simulink model "W15_Road_Side_Parking_cs"  (R2019a)
settings: Solver=ode5  StartTime=0.0  StopTime=inf  FixedStep=1/20  RelTol=1e-3
PreLoadFcn:
  | mbxruntime.callbacks.PreLoadFcn(bdroot);
PostLoadFcn:
  | mbxruntime.callbacks.PostLoadFcn(bdroot);
InitFcn:
  | mbxruntime.callbacks.InitFcn(bdroot);
StartFcn:
  | mbxruntime.callbacks.StartFcn(bdroot);
StopFcn:
  | mbxruntime.callbacks.StopFcn(bdroot);
model workspace: external: MAT-File .\W15_Road_Side_Parking_cs_hws.mat (data not in the file)
undefined symbols (not defined in the file or in its folder): DiscIntNeverNeededParam, mbxruntime, W15_Road_Side_Parking_cs_0e866b970dd74d99, W15_Road_Side_Parking_cs_0f148a56f75f3276, W15_Road_Side_Parking_cs_17cd01741fd6f084, W15_Road_Side_Parking_cs_18be040ea5165f26, W15_Road_Side_Parking_cs_18f6c04aadf175ba, W15_Road_Side_Parking_cs_1923d3106c1c637d, W15_Road_Side_Parking_cs_1b5a4544d45624a7, W15_Road_Side_Parking_cs_1b6c0c20ec73a43a, W15_Road_Side_Parking_cs_2b0ebcffe59377d8, W15_Road_Side_Parking_cs_31ff6997c9af0f31, W15_Road_Side_Parking_cs_38fd1df42ec62113, W15_Road_Side_Parking_cs_3b33461cc0923d5a, W15_Road_Side_Parking_cs_3fb29b605fd2446e, W15_Road_Side_Parking_cs_415727a4762a2f3b, W15_Road_Side_Parking_cs_42e4989f077d83f1, W15_Road_Side_Parking_cs_437d21a73ee2a604, W15_Road_Side_Parking_cs_438c4f208d99b00a, W15_Road_Side_Parking_cs_43af58d29723f162, W15_Road_Side_Parking_cs_46e56dcb0f84eb7a, W15_Road_Side_Parking_cs_4b469b712dfdc78c, W15_Road_Side_Parking_cs_52f5bda9b370cee6, W15_Road_Side_Parking_cs_53d6cec13a681255, W15_Road_Side_Parking_cs_55198fcb4bd3c3cf, W15_Road_Side_Parking_cs_55651d2ac6314b5a, W15_Road_Side_Parking_cs_566668cc8d93055a, W15_Road_Side_Parking_cs_5685e0897f4c48c1, W15_Road_Side_Parking_cs_59579d35ff31c10a, W15_Road_Side_Parking_cs_59ff7782c70c6b28, W15_Road_Side_Parking_cs_5bf98cb8ec781366, W15_Road_Side_Parking_cs_5f42887855dc872c, W15_Road_Side_Parking_cs_6189064c2a21a5a0, W15_Road_Side_Parking_cs_6a2215e73604bb67, W15_Road_Side_Parking_cs_71a8b3b44613f615, W15_Road_Side_Parking_cs_71c6ac7bb3dca246, W15_Road_Side_Parking_cs_71fd76710240543d, W15_Road_Side_Parking_cs_745c3945ff638ec3, W15_Road_Side_Parking_cs_7a6c1e7b0eb6c7b9, W15_Road_Side_Parking_cs_85e359d40c717561, W15_Road_Side_Parking_cs_8b52fd1869158bfe, W15_Road_Side_Parking_cs_8bff9458d942351f, W15_Road_Side_Parking_cs_8c4b607c5829f2a9, W15_Road_Side_Parking_cs_8f8185f5cf144aaf, W15_Road_Side_Parking_cs_93695886b652e87b, W15_Road_Side_Parking_cs_97c6d597a0216a81, W15_Road_Side_Parking_cs_9b084c5c3aa0b401, W15_Road_Side_Parking_cs_9c145665a20a76f3, W15_Road_Side_Parking_cs_9dd5e77a4f43e96a, W15_Road_Side_Parking_cs_a44a67f2721d9815, W15_Road_Side_Parking_cs_a5d6455b7e6bd0b2, W15_Road_Side_Parking_cs_a72a872bc8c596f9, W15_Road_Side_Parking_cs_ab6502bd2087c801, W15_Road_Side_Parking_cs_ad8c05542c501359, W15_Road_Side_Parking_cs_ae0701bb52210b9e, W15_Road_Side_Parking_cs_b19e05410c02f142, W15_Road_Side_Parking_cs_b31b08a7b69b63e6, W15_Road_Side_Parking_cs_b3b5053d85c8642b, W15_Road_Side_Parking_cs_bbd847625a8d6d3d, W15_Road_Side_Parking_cs_bc9116e6f1ce847b ... (+26)
libraries: adeye_lib x37, PreScanSimulinkLibrary x28, PreScanUsefulBlocks x1
(part 2 of 10)

== system W15_Road_Side_Parking_cs/AIR_3 ==
  Sensor : S-Function  FunctionName=sfun_AIRSensor  Parameters=mbxruntime.parameters.convert(detectableObjects), mbxruntime.parameters.convert(sensorID), mbxruntime.parameters.convert(timestep)  SFunctionDeploymentMode=off  EnableBusSupport=off  mask(PreScan Source Block: Actor Independent Receiver (AIR)){detectableObjects=1, sensorID=3596, timestep=1/20}
      mask prompts: detectableObjects "Max detectable objects"; sensorID "Sensor ID"; timestep "MATLAB timestep:"
      mask help:
      | The Actor Information Receiver sensor provides a fast, simple and generic detection solution which is not tied up to a specific technology. The AIR detects the intersection point of the bounding box with the straight line from the sensor axis system to the middle of the bounding box.
      |
      | For more information, please click Help.
      mask Help: eval('openHelp(413)')
      mask Display: image(imread('AIR.png'))
  AIR_3 : Outport  Tag=outport/AIR  OutDataTypeStr=Bus: PRESCAN_AIRSENSORMESSAGE  PortDimensions=1  SampleTime=1/20
  wires:
  Sensor/1 -> AIR_3/1

== system W15_Road_Side_Parking_cs/AIR_4 ==
  Sensor : S-Function  FunctionName=sfun_AIRSensor  Parameters=mbxruntime.parameters.convert(detectableObjects), mbxruntime.parameters.convert(sensorID), mbxruntime.parameters.convert(timestep)  SFunctionDeploymentMode=off  EnableBusSupport=off  mask(PreScan Source Block: Actor Independent Receiver (AIR)){detectableObjects=1, sensorID=3598, timestep=1/20}
      mask prompts: detectableObjects "Max detectable objects"; sensorID "Sensor ID"; timestep "MATLAB timestep:"
      mask help:
      | The Actor Information Receiver sensor provides a fast, simple and generic detection solution which is not tied up to a specific technology. The AIR detects the intersection point of the bounding box with the straight line from the sensor axis system to the middle of the bounding box.
      |
      | For more information, please click Help.
      mask Help: eval('openHelp(413)')
      mask Display: image(imread('AIR.png'))
  AIR_4 : Outport  Tag=outport/AIR  OutDataTypeStr=Bus: PRESCAN_AIRSENSORMESSAGE  PortDimensions=1  SampleTime=1/20
  wires:
  Sensor/1 -> AIR_4/1

== system W15_Road_Side_Parking_cs/AIR_5 ==
  Sensor : S-Function  FunctionName=sfun_AIRSensor  Parameters=mbxruntime.parameters.convert(detectableObjects), mbxruntime.parameters.convert(sensorID), mbxruntime.parameters.convert(timestep)  SFunctionDeploymentMode=off  EnableBusSupport=off  mask(PreScan Source Block: Actor Independent Receiver (AIR)){detectableObjects=1, sensorID=3600, timestep=1/20}
      mask prompts: detectableObjects "Max detectable objects"; sensorID "Sensor ID"; timestep "MATLAB timestep:"
      mask help:
      | The Actor Information Receiver sensor provides a fast, simple and generic detection solution which is not tied up to a specific technology. The AIR detects the intersection point of the bounding box with the straight line from the sensor axis system to the middle of the bounding box.
      |
      | For more information, please click Help.
      mask Help: eval('openHelp(413)')
      mask Display: image(imread('AIR.png'))
  AIR_5 : Outport  Tag=outport/AIR  OutDataTypeStr=Bus: PRESCAN_AIRSENSORMESSAGE  PortDimensions=1  SampleTime=1/20
  wires:
  Sensor/1 -> AIR_5/1

== system W15_Road_Side_Parking_cs/AIR_6 ==
  Sensor : S-Function  FunctionName=sfun_AIRSensor  Parameters=mbxruntime.parameters.convert(detectableObjects), mbxruntime.parameters.convert(sensorID), mbxruntime.parameters.convert(timestep)  SFunctionDeploymentMode=off  EnableBusSupport=off  mask(PreScan Source Block: Actor Independent Receiver (AIR)){detectableObjects=1, sensorID=3960, timestep=1/20}
      mask prompts: detectableObjects "Max detectable objects"; sensorID "Sensor ID"; timestep "MATLAB timestep:"
      mask help:
      | The Actor Information Receiver sensor provides a fast, simple and generic detection solution which is not tied up to a specific technology. The AIR detects the intersection point of the bounding box with the straight line from the sensor axis system to the middle of the bounding box.
      |
      | For more information, please click Help.
      mask Help: eval('openHelp(413)')
      mask Display: image(imread('AIR.png'))
  AIR_6 : Outport  Tag=outport/AIR  OutDataTypeStr=Bus: PRESCAN_AIRSENSORMESSAGE  PortDimensions=1  SampleTime=1/20
  wires:
  Sensor/1 -> AIR_6/1

== system W15_Road_Side_Parking_cs/AIR_7 ==
  Sensor : S-Function  FunctionName=sfun_AIRSensor  Parameters=mbxruntime.parameters.convert(detectableObjects), mbxruntime.parameters.convert(sensorID), mbxruntime.parameters.convert(timestep)  SFunctionDeploymentMode=off  EnableBusSupport=off  mask(PreScan Source Block: Actor Independent Receiver (AIR)){detectableObjects=1, sensorID=3962, timestep=1/20}
      mask prompts: detectableObjects "Max detectable objects"; sensorID "Sensor ID"; timestep "MATLAB timestep:"
      mask help:
      | The Actor Information Receiver sensor provides a fast, simple and generic detection solution which is not tied up to a specific technology. The AIR detects the intersection point of the bounding box with the straight line from the sensor axis system to the middle of the bounding box.
      |
      | For more information, please click Help.
      mask Help: eval('openHelp(413)')
      mask Display: image(imread('AIR.png'))
  AIR_7 : Outport  Tag=outport/AIR  OutDataTypeStr=Bus: PRESCAN_AIRSENSORMESSAGE  PortDimensions=1  SampleTime=1/20
  wires:
  Sensor/1 -> AIR_7/1

== system W15_Road_Side_Parking_cs/AIR_8 ==
  Sensor : S-Function  FunctionName=sfun_AIRSensor  Parameters=mbxruntime.parameters.convert(detectableObjects), mbxruntime.parameters.convert(sensorID), mbxruntime.parameters.convert(timestep)  SFunctionDeploymentMode=off  EnableBusSupport=off  mask(PreScan Source Block: Actor Independent Receiver (AIR)){detectableObjects=1, sensorID=3964, timestep=1/20}
      mask prompts: detectableObjects "Max detectable objects"; sensorID "Sensor ID"; timestep "MATLAB timestep:"
      mask help:
      | The Actor Information Receiver sensor provides a fast, simple and generic detection solution which is not tied up to a specific technology. The AIR detects the intersection point of the bounding box with the straight line from the sensor axis system to the middle of the bounding box.
      |
      | For more information, please click Help.
      mask Help: eval('openHelp(413)')
      mask Display: image(imread('AIR.png'))
  AIR_8 : Outport  Tag=outport/AIR  OutDataTypeStr=Bus: PRESCAN_AIRSENSORMESSAGE  PortDimensions=1  SampleTime=1/20
  wires:
  Sensor/1 -> AIR_8/1

== system W15_Road_Side_Parking_cs/AIR_9 ==
  Sensor : S-Function  FunctionName=sfun_AIRSensor  Parameters=mbxruntime.parameters.convert(detectableObjects), mbxruntime.parameters.convert(sensorID), mbxruntime.parameters.convert(timestep)  SFunctionDeploymentMode=off  EnableBusSupport=off  mask(PreScan Source Block: Actor Independent Receiver (AIR)){detectableObjects=1, sensorID=3966, timestep=1/20}
      mask prompts: detectableObjects "Max detectable objects"; sensorID "Sensor ID"; timestep "MATLAB timestep:"
      mask help:
      | The Actor Information Receiver sensor provides a fast, simple and generic detection solution which is not tied up to a specific technology. The AIR detects the intersection point of the bounding box with the straight line from the sensor axis system to the middle of the bounding box.
      |
      | For more information, please click Help.
      mask Help: eval('openHelp(413)')
      mask Display: image(imread('AIR.png'))
  AIR_9 : Outport  Tag=outport/AIR  OutDataTypeStr=Bus: PRESCAN_AIRSENSORMESSAGE  PortDimensions=1  SampleTime=1/20
  wires:
  Sensor/1 -> AIR_9/1

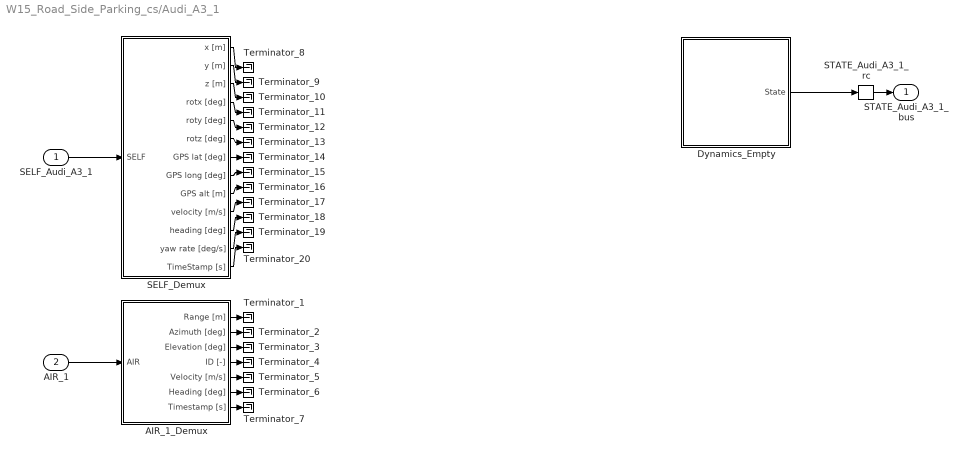
== system W15_Road_Side_Parking_cs/Audi_A3_1 ==
  SELF_Audi_A3_1 : Inport  Tag=inport/SelfPort  OutDataTypeStr=Bus: PRESCAN_SELFSENSORDATA  PortDimensions=1  SampleTime=1/20  BusOutputAsStruct=on
  AIR_1 : Inport  Tag=inport/AIR  Port=2  OutDataTypeStr=Bus: PRESCAN_AIRSENSORMESSAGE  PortDimensions=1  SampleTime=1/20  BusOutputAsStruct=on
  AIR_1_Demux : Subsystem  Tag=demux/AIR  mask(PreScan Demux Block: AIR){DetectionType=BBox, detectableObjects=1}
      mask prompts: DetectionType "Detection Type"; detectableObjects "Max. detectable objects"
      mask help:
      | The Actor Information Receiver sensor provides a fast, simple and generic detection solution which is not tied up to a specific technology and can be used for scenarios in which a simple sensor is needed.
      |
      | For more information, please click Help.
      mask init:
      | switch DetectionType
      |     case 1
      |         DetectionTypeStr = 'Center';
      |     case 2
      |         DetectionTypeStr = 'BBox';
      |     case 3
      |         DetectionTypeStr = 'CoG';
      |     otherwise
      |         DetectionTypeStr = 'Unknown';
      | end
      settings: DeleteFcn=PreScanBlockDeleteFcn;
      mask Help: eval('openHelp(413)')
      mask TypeOptions DetectionType: Center | BBox | CoG
      mask Display:
      | disp(char('Det. type:         ',['{\it',DetectionTypeStr,'}']),'texmode','on')
      | port_label('output',1,'Range [m]')
      | port_label('output',2,'{\theta} [deg]','texmode','on')
      | port_label('output',3,'{\phi} [deg]','texmode','on')
      | port_label('output',4,'ID [-]','texmode','on')
      | port_label('output',5,'Velocity [m/s]','texmode','on')
      | port_label('output',6,'Heading [deg]','texmode','on')
      | port_label('output',7,'Timestamp [s]','texmode','on')
  Dynamics_Empty : Subsystem  Tag=Dynamics_Empty
      mask Help: eval('openHelp(202)')
      mask Display: port_label('output', 1, 'State');text(0,0,' Empty\n')
  SELF_Demux : Subsystem  Tag=demux/SelfPort  mask(PreScan Demux Block:){}
      mask help:
      | The SELF port shows (state) information of the actor itself. The outputs are position in the experiment's axis system and the GPS coordinates, and the object's absolute velocity and compass heading.
      |
      | For more information, please click Help.
      settings: DeleteFcn=PreScanBlockDeleteFcn;
      mask Help: eval('openHelp(462)')
      mask Display:
      | port_label('output',1,'x [m]')
      | port_label('output',2,'y [m]')
      | port_label('output',3,'z [m]','texmode','on')
      | port_label('output',4,'Rotx [deg]','texmode','on')
      | port_label('output',5,'Roty [deg]','texmode','on')
      | port_label('output',6,'Rotz [deg]','texmode','on')
      | port_label('output',7,'GPS lat [deg]','texmode','on')
      | port_label('output',8,'GPS long [deg]','texmode','on')
      | port_label('output',9,'GPS alt [m]','texmode','on')
      | port_label('output',10,'Velocity [m/s]')
      | port_label('output',11,'Heading [deg]')
      | port_label('output',12,'Yaw rate [deg/s]')
      | port_label('output',13,'Timestamp [s]')
  STATE_Audi_A3_1_rc : RateTransition  Tag=mux_rc/StatePort  OutPortSampleTimeOpt=Inherit
  Terminator_{1..20} (20 alike) : Terminator
  STATE_Audi_A3_1_bus : Outport  Tag=outport/StatePort  OutDataTypeStr=Bus: PRESCAN_STATEACTUATORDATA  PortDimensions=1  SampleTime=1/20
  wires:
  STATE_Audi_A3_1_rc/1 -> STATE_Audi_A3_1_bus/1
  SELF_Audi_A3_1/1 -> SELF_Demux/1(SELF)
  AIR_1/1 -> AIR_1_Demux/1(AIR)
  Dynamics_Empty/1(State) -> STATE_Audi_A3_1_rc/1
  AIR_1_Demux/1(Range [m]) -> Terminator_1/1
  AIR_1_Demux/2(Azimuth [deg]) -> Terminator_2/1
  AIR_1_Demux/3(Elevation [deg]) -> Terminator_3/1
  AIR_1_Demux/4(ID [-]) -> Terminator_4/1
  AIR_1_Demux/5(Velocity [m/s]) -> Terminator_5/1
  AIR_1_Demux/6(Heading [deg]) -> Terminator_6/1
  AIR_1_Demux/7(Timestamp [s]) -> Terminator_7/1
  SELF_Demux/1(x [m]) -> Terminator_8/1
  SELF_Demux/2(y [m]) -> Terminator_9/1
  SELF_Demux/3(z [m]) -> Terminator_10/1
  SELF_Demux/4(rotx [deg]) -> Terminator_11/1
  SELF_Demux/5(roty [deg]) -> Terminator_12/1
  SELF_Demux/6(rotz [deg]) -> Terminator_13/1
  SELF_Demux/7(GPS lat [deg]) -> Terminator_14/1
  SELF_Demux/8(GPS long [deg]) -> Terminator_15/1
  SELF_Demux/9(GPS alt [m]) -> Terminator_16/1
  SELF_Demux/10(velocity [m/s]) -> Terminator_17/1
  SELF_Demux/11(heading [deg]) -> Terminator_18/1
  SELF_Demux/12(yaw rate [deg/s]) -> Terminator_19/1
  SELF_Demux/13(TimeStamp [s]) -> Terminator_20/1

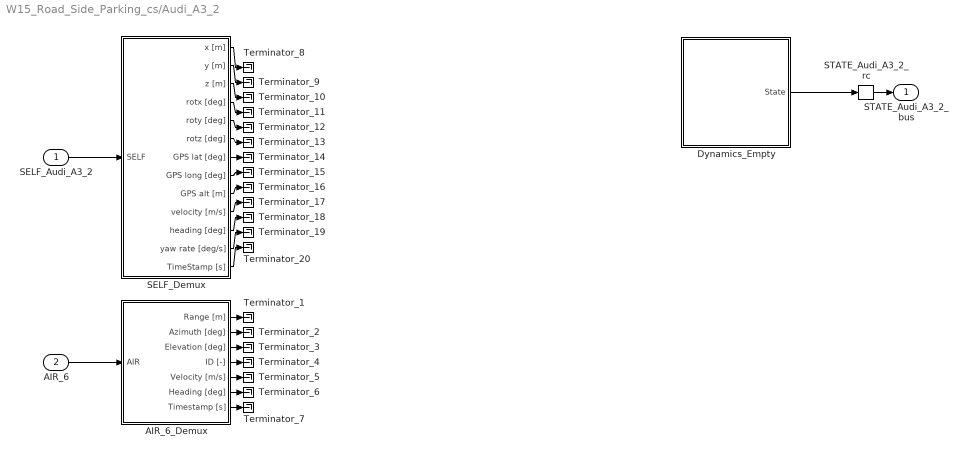
== system W15_Road_Side_Parking_cs/Audi_A3_2 ==
  SELF_Audi_A3_2 : Inport  Tag=inport/SelfPort  OutDataTypeStr=Bus: PRESCAN_SELFSENSORDATA  PortDimensions=1  SampleTime=1/20  BusOutputAsStruct=on
  AIR_6 : Inport  Tag=inport/AIR  Port=2  OutDataTypeStr=Bus: PRESCAN_AIRSENSORMESSAGE  PortDimensions=1  SampleTime=1/20  BusOutputAsStruct=on
  AIR_6_Demux : Subsystem  Tag=demux/AIR  mask(PreScan Demux Block: AIR){DetectionType=BBox, detectableObjects=1}
      mask prompts: DetectionType "Detection Type"; detectableObjects "Max. detectable objects"
      mask help:
      | The Actor Information Receiver sensor provides a fast, simple and generic detection solution which is not tied up to a specific technology and can be used for scenarios in which a simple sensor is needed.
      |
      | For more information, please click Help.
      mask init: same as W15_Road_Side_Parking_cs/Audi_A3_1/AIR_1_Demux
      settings: DeleteFcn=PreScanBlockDeleteFcn;
      mask Help: eval('openHelp(413)')
      mask TypeOptions DetectionType: Center | BBox | CoG
      mask Display:
      | disp(char('Det. type:         ',['{\it',DetectionTypeStr,'}']),'texmode','on')
      | port_label('output',1,'Range [m]')
      | port_label('output',2,'{\theta} [deg]','texmode','on')
      | port_label('output',3,'{\phi} [deg]','texmode','on')
      | port_label('output',4,'ID [-]','texmode','on')
      | port_label('output',5,'Velocity [m/s]','texmode','on')
      | port_label('output',6,'Heading [deg]','texmode','on')
      | port_label('output',7,'Timestamp [s]','texmode','on')
  Dynamics_Empty : Subsystem  Tag=Dynamics_Empty
      mask Help: eval('openHelp(202)')
      mask Display: port_label('output', 1, 'State');text(0,0,' Empty\n')
  SELF_Demux : Subsystem  Tag=demux/SelfPort  mask(PreScan Demux Block:){}
      mask help:
      | The SELF port shows (state) information of the actor itself. The outputs are position in the experiment's axis system and the GPS coordinates, and the object's absolute velocity and compass heading.
      |
      | For more information, please click Help.
      settings: DeleteFcn=PreScanBlockDeleteFcn;
      mask Help: eval('openHelp(462)')
      mask Display:
      | port_label('output',1,'x [m]')
      | port_label('output',2,'y [m]')
      | port_label('output',3,'z [m]','texmode','on')
      | port_label('output',4,'Rotx [deg]','texmode','on')
      | port_label('output',5,'Roty [deg]','texmode','on')
      | port_label('output',6,'Rotz [deg]','texmode','on')
      | port_label('output',7,'GPS lat [deg]','texmode','on')
      | port_label('output',8,'GPS long [deg]','texmode','on')
      | port_label('output',9,'GPS alt [m]','texmode','on')
      | port_label('output',10,'Velocity [m/s]')
      | port_label('output',11,'Heading [deg]')
      | port_label('output',12,'Yaw rate [deg/s]')
      | port_label('output',13,'Timestamp [s]')
  STATE_Audi_A3_2_rc : RateTransition  Tag=mux_rc/StatePort  OutPortSampleTimeOpt=Inherit
  Terminator_{1..20} (20 alike) : Terminator
  STATE_Audi_A3_2_bus : Outport  Tag=outport/StatePort  OutDataTypeStr=Bus: PRESCAN_STATEACTUATORDATA  PortDimensions=1  SampleTime=1/20
  wires:
  STATE_Audi_A3_2_rc/1 -> STATE_Audi_A3_2_bus/1
  SELF_Audi_A3_2/1 -> SELF_Demux/1(SELF)
  AIR_6/1 -> AIR_6_Demux/1(AIR)
  Dynamics_Empty/1(State) -> STATE_Audi_A3_2_rc/1
  AIR_6_Demux/1(Range [m]) -> Terminator_1/1
  AIR_6_Demux/2(Azimuth [deg]) -> Terminator_2/1
  AIR_6_Demux/3(Elevation [deg]) -> Terminator_3/1
  AIR_6_Demux/4(ID [-]) -> Terminator_4/1
  AIR_6_Demux/5(Velocity [m/s]) -> Terminator_5/1
  AIR_6_Demux/6(Heading [deg]) -> Terminator_6/1
  AIR_6_Demux/7(Timestamp [s]) -> Terminator_7/1
  SELF_Demux/1(x [m]) -> Terminator_8/1
  SELF_Demux/2(y [m]) -> Terminator_9/1
  SELF_Demux/3(z [m]) -> Terminator_10/1
  SELF_Demux/4(rotx [deg]) -> Terminator_11/1
  SELF_Demux/5(roty [deg]) -> Terminator_12/1
  SELF_Demux/6(rotz [deg]) -> Terminator_13/1
  SELF_Demux/7(GPS lat [deg]) -> Terminator_14/1
  SELF_Demux/8(GPS long [deg]) -> Terminator_15/1
  SELF_Demux/9(GPS alt [m]) -> Terminator_16/1
  SELF_Demux/10(velocity [m/s]) -> Terminator_17/1
  SELF_Demux/11(heading [deg]) -> Terminator_18/1
  SELF_Demux/12(yaw rate [deg/s]) -> Terminator_19/1
  SELF_Demux/13(TimeStamp [s]) -> Terminator_20/1

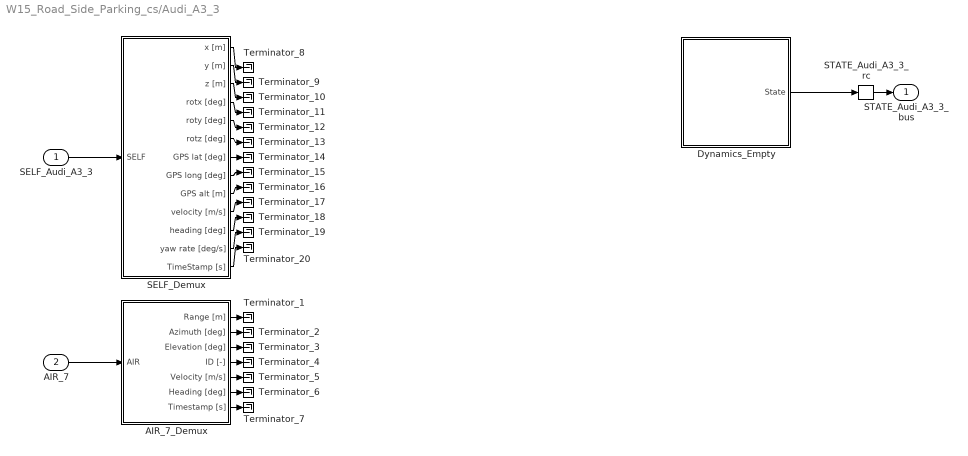
== system W15_Road_Side_Parking_cs/Audi_A3_3 ==
  SELF_Audi_A3_3 : Inport  Tag=inport/SelfPort  OutDataTypeStr=Bus: PRESCAN_SELFSENSORDATA  PortDimensions=1  SampleTime=1/20  BusOutputAsStruct=on
  AIR_7 : Inport  Tag=inport/AIR  Port=2  OutDataTypeStr=Bus: PRESCAN_AIRSENSORMESSAGE  PortDimensions=1  SampleTime=1/20  BusOutputAsStruct=on
  AIR_7_Demux : Subsystem  Tag=demux/AIR  mask(PreScan Demux Block: AIR){DetectionType=BBox, detectableObjects=1}
      mask prompts: DetectionType "Detection Type"; detectableObjects "Max. detectable objects"
      mask help:
      | The Actor Information Receiver sensor provides a fast, simple and generic detection solution which is not tied up to a specific technology and can be used for scenarios in which a simple sensor is needed.
      |
      | For more information, please click Help.
      mask init: same as W15_Road_Side_Parking_cs/Audi_A3_1/AIR_1_Demux
      settings: DeleteFcn=PreScanBlockDeleteFcn;
      mask Help: eval('openHelp(413)')
      mask TypeOptions DetectionType: Center | BBox | CoG
      mask Display:
      | disp(char('Det. type:         ',['{\it',DetectionTypeStr,'}']),'texmode','on')
      | port_label('output',1,'Range [m]')
      | port_label('output',2,'{\theta} [deg]','texmode','on')
      | port_label('output',3,'{\phi} [deg]','texmode','on')
      | port_label('output',4,'ID [-]','texmode','on')
      | port_label('output',5,'Velocity [m/s]','texmode','on')
      | port_label('output',6,'Heading [deg]','texmode','on')
      | port_label('output',7,'Timestamp [s]','texmode','on')
  Dynamics_Empty : Subsystem  Tag=Dynamics_Empty
      mask Help: eval('openHelp(202)')
      mask Display: port_label('output', 1, 'State');text(0,0,' Empty\n')
  SELF_Demux : Subsystem  Tag=demux/SelfPort  mask(PreScan Demux Block:){}
      mask help:
      | The SELF port shows (state) information of the actor itself. The outputs are position in the experiment's axis system and the GPS coordinates, and the object's absolute velocity and compass heading.
      |
      | For more information, please click Help.
      settings: DeleteFcn=PreScanBlockDeleteFcn;
      mask Help: eval('openHelp(462)')
      mask Display:
      | port_label('output',1,'x [m]')
      | port_label('output',2,'y [m]')
      | port_label('output',3,'z [m]','texmode','on')
      | port_label('output',4,'Rotx [deg]','texmode','on')
      | port_label('output',5,'Roty [deg]','texmode','on')
      | port_label('output',6,'Rotz [deg]','texmode','on')
      | port_label('output',7,'GPS lat [deg]','texmode','on')
      | port_label('output',8,'GPS long [deg]','texmode','on')
      | port_label('output',9,'GPS alt [m]','texmode','on')
      | port_label('output',10,'Velocity [m/s]')
      | port_label('output',11,'Heading [deg]')
      | port_label('output',12,'Yaw rate [deg/s]')
      | port_label('output',13,'Timestamp [s]')
  STATE_Audi_A3_3_rc : RateTransition  Tag=mux_rc/StatePort  OutPortSampleTimeOpt=Inherit
  Terminator_{1..20} (20 alike) : Terminator
  STATE_Audi_A3_3_bus : Outport  Tag=outport/StatePort  OutDataTypeStr=Bus: PRESCAN_STATEACTUATORDATA  PortDimensions=1  SampleTime=1/20
  wires:
  STATE_Audi_A3_3_rc/1 -> STATE_Audi_A3_3_bus/1
  SELF_Audi_A3_3/1 -> SELF_Demux/1(SELF)
  AIR_7/1 -> AIR_7_Demux/1(AIR)
  Dynamics_Empty/1(State) -> STATE_Audi_A3_3_rc/1
  AIR_7_Demux/1(Range [m]) -> Terminator_1/1
  AIR_7_Demux/2(Azimuth [deg]) -> Terminator_2/1
  AIR_7_Demux/3(Elevation [deg]) -> Terminator_3/1
  AIR_7_Demux/4(ID [-]) -> Terminator_4/1
  AIR_7_Demux/5(Velocity [m/s]) -> Terminator_5/1
  AIR_7_Demux/6(Heading [deg]) -> Terminator_6/1
  AIR_7_Demux/7(Timestamp [s]) -> Terminator_7/1
  SELF_Demux/1(x [m]) -> Terminator_8/1
  SELF_Demux/2(y [m]) -> Terminator_9/1
  SELF_Demux/3(z [m]) -> Terminator_10/1
  SELF_Demux/4(rotx [deg]) -> Terminator_11/1
  SELF_Demux/5(roty [deg]) -> Terminator_12/1
  SELF_Demux/6(rotz [deg]) -> Terminator_13/1
  SELF_Demux/7(GPS lat [deg]) -> Terminator_14/1
  SELF_Demux/8(GPS long [deg]) -> Terminator_15/1
  SELF_Demux/9(GPS alt [m]) -> Terminator_16/1
  SELF_Demux/10(velocity [m/s]) -> Terminator_17/1
  SELF_Demux/11(heading [deg]) -> Terminator_18/1
  SELF_Demux/12(yaw rate [deg/s]) -> Terminator_19/1
  SELF_Demux/13(TimeStamp [s]) -> Terminator_20/1

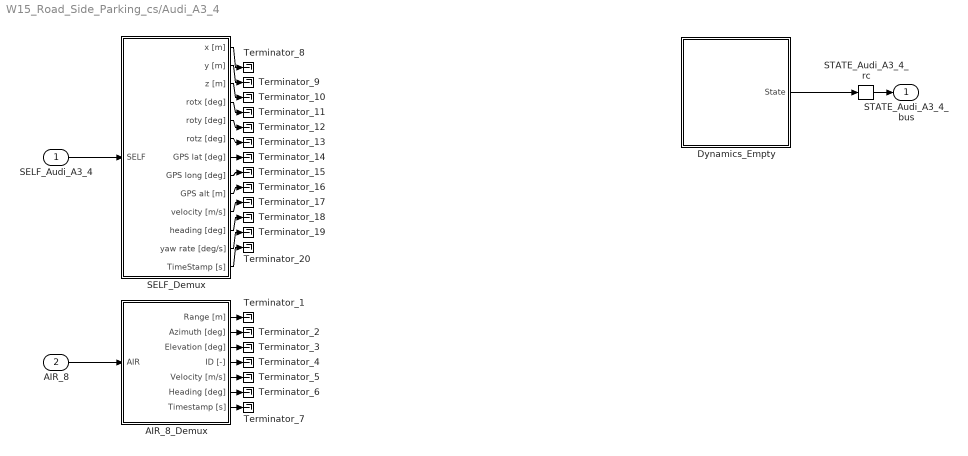
== system W15_Road_Side_Parking_cs/Audi_A3_4 ==
  SELF_Audi_A3_4 : Inport  Tag=inport/SelfPort  OutDataTypeStr=Bus: PRESCAN_SELFSENSORDATA  PortDimensions=1  SampleTime=1/20  BusOutputAsStruct=on
  AIR_8 : Inport  Tag=inport/AIR  Port=2  OutDataTypeStr=Bus: PRESCAN_AIRSENSORMESSAGE  PortDimensions=1  SampleTime=1/20  BusOutputAsStruct=on
  AIR_8_Demux : Subsystem  Tag=demux/AIR  mask(PreScan Demux Block: AIR){DetectionType=BBox, detectableObjects=1}
      mask prompts: DetectionType "Detection Type"; detectableObjects "Max. detectable objects"
      mask help:
      | The Actor Information Receiver sensor provides a fast, simple and generic detection solution which is not tied up to a specific technology and can be used for scenarios in which a simple sensor is needed.
      |
      | For more information, please click Help.
      mask init: same as W15_Road_Side_Parking_cs/Audi_A3_1/AIR_1_Demux
      settings: DeleteFcn=PreScanBlockDeleteFcn;
      mask Help: eval('openHelp(413)')
      mask TypeOptions DetectionType: Center | BBox | CoG
      mask Display:
      | disp(char('Det. type:         ',['{\it',DetectionTypeStr,'}']),'texmode','on')
      | port_label('output',1,'Range [m]')
      | port_label('output',2,'{\theta} [deg]','texmode','on')
      | port_label('output',3,'{\phi} [deg]','texmode','on')
      | port_label('output',4,'ID [-]','texmode','on')
      | port_label('output',5,'Velocity [m/s]','texmode','on')
      | port_label('output',6,'Heading [deg]','texmode','on')
      | port_label('output',7,'Timestamp [s]','texmode','on')
  Dynamics_Empty : Subsystem  Tag=Dynamics_Empty
      mask Help: eval('openHelp(202)')
      mask Display: port_label('output', 1, 'State');text(0,0,' Empty\n')
  SELF_Demux : Subsystem  Tag=demux/SelfPort  mask(PreScan Demux Block:){}
      mask help:
      | The SELF port shows (state) information of the actor itself. The outputs are position in the experiment's axis system and the GPS coordinates, and the object's absolute velocity and compass heading.
      |
      | For more information, please click Help.
      settings: DeleteFcn=PreScanBlockDeleteFcn;
      mask Help: eval('openHelp(462)')
      mask Display:
      | port_label('output',1,'x [m]')
      | port_label('output',2,'y [m]')
      | port_label('output',3,'z [m]','texmode','on')
      | port_label('output',4,'Rotx [deg]','texmode','on')
      | port_label('output',5,'Roty [deg]','texmode','on')
      | port_label('output',6,'Rotz [deg]','texmode','on')
      | port_label('output',7,'GPS lat [deg]','texmode','on')
      | port_label('output',8,'GPS long [deg]','texmode','on')
      | port_label('output',9,'GPS alt [m]','texmode','on')
      | port_label('output',10,'Velocity [m/s]')
      | port_label('output',11,'Heading [deg]')
      | port_label('output',12,'Yaw rate [deg/s]')
      | port_label('output',13,'Timestamp [s]')
  STATE_Audi_A3_4_rc : RateTransition  Tag=mux_rc/StatePort  OutPortSampleTimeOpt=Inherit
  Terminator_{1..20} (20 alike) : Terminator
  STATE_Audi_A3_4_bus : Outport  Tag=outport/StatePort  OutDataTypeStr=Bus: PRESCAN_STATEACTUATORDATA  PortDimensions=1  SampleTime=1/20
  wires:
  STATE_Audi_A3_4_rc/1 -> STATE_Audi_A3_4_bus/1
  SELF_Audi_A3_4/1 -> SELF_Demux/1(SELF)
  AIR_8/1 -> AIR_8_Demux/1(AIR)
  Dynamics_Empty/1(State) -> STATE_Audi_A3_4_rc/1
  AIR_8_Demux/1(Range [m]) -> Terminator_1/1
  AIR_8_Demux/2(Azimuth [deg]) -> Terminator_2/1
  AIR_8_Demux/3(Elevation [deg]) -> Terminator_3/1
  AIR_8_Demux/4(ID [-]) -> Terminator_4/1
  AIR_8_Demux/5(Velocity [m/s]) -> Terminator_5/1
  AIR_8_Demux/6(Heading [deg]) -> Terminator_6/1
  AIR_8_Demux/7(Timestamp [s]) -> Terminator_7/1
  SELF_Demux/1(x [m]) -> Terminator_8/1
  SELF_Demux/2(y [m]) -> Terminator_9/1
  SELF_Demux/3(z [m]) -> Terminator_10/1
  SELF_Demux/4(rotx [deg]) -> Terminator_11/1
  SELF_Demux/5(roty [deg]) -> Terminator_12/1
  SELF_Demux/6(rotz [deg]) -> Terminator_13/1
  SELF_Demux/7(GPS lat [deg]) -> Terminator_14/1
  SELF_Demux/8(GPS long [deg]) -> Terminator_15/1
  SELF_Demux/9(GPS alt [m]) -> Terminator_16/1
  SELF_Demux/10(velocity [m/s]) -> Terminator_17/1
  SELF_Demux/11(heading [deg]) -> Terminator_18/1
  SELF_Demux/12(yaw rate [deg/s]) -> Terminator_19/1
  SELF_Demux/13(TimeStamp [s]) -> Terminator_20/1

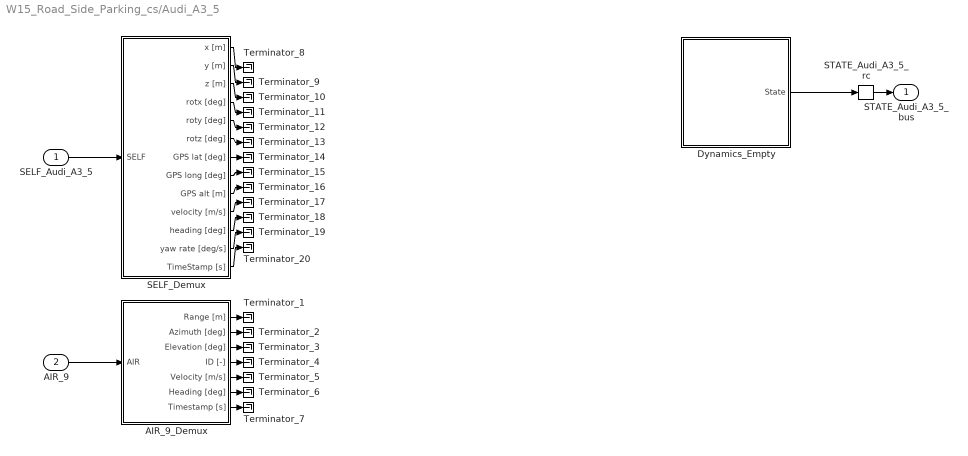
== system W15_Road_Side_Parking_cs/Audi_A3_5 ==
  SELF_Audi_A3_5 : Inport  Tag=inport/SelfPort  OutDataTypeStr=Bus: PRESCAN_SELFSENSORDATA  PortDimensions=1  SampleTime=1/20  BusOutputAsStruct=on
  AIR_9 : Inport  Tag=inport/AIR  Port=2  OutDataTypeStr=Bus: PRESCAN_AIRSENSORMESSAGE  PortDimensions=1  SampleTime=1/20  BusOutputAsStruct=on
  AIR_9_Demux : Subsystem  Tag=demux/AIR  mask(PreScan Demux Block: AIR){DetectionType=BBox, detectableObjects=1}
      mask prompts: DetectionType "Detection Type"; detectableObjects "Max. detectable objects"
      mask help:
      | The Actor Information Receiver sensor provides a fast, simple and generic detection solution which is not tied up to a specific technology and can be used for scenarios in which a simple sensor is needed.
      |
      | For more information, please click Help.
      mask init: same as W15_Road_Side_Parking_cs/Audi_A3_1/AIR_1_Demux
      settings: DeleteFcn=PreScanBlockDeleteFcn;
      mask Help: eval('openHelp(413)')
      mask TypeOptions DetectionType: Center | BBox | CoG
      mask Display:
      | disp(char('Det. type:         ',['{\it',DetectionTypeStr,'}']),'texmode','on')
      | port_label('output',1,'Range [m]')
      | port_label('output',2,'{\theta} [deg]','texmode','on')
      | port_label('output',3,'{\phi} [deg]','texmode','on')
      | port_label('output',4,'ID [-]','texmode','on')
      | port_label('output',5,'Velocity [m/s]','texmode','on')
      | port_label('output',6,'Heading [deg]','texmode','on')
      | port_label('output',7,'Timestamp [s]','texmode','on')
  Dynamics_Empty : Subsystem  Tag=Dynamics_Empty
      mask Help: eval('openHelp(202)')
      mask Display: port_label('output', 1, 'State');text(0,0,' Empty\n')
  SELF_Demux : Subsystem  Tag=demux/SelfPort  mask(PreScan Demux Block:){}
      mask help:
      | The SELF port shows (state) information of the actor itself. The outputs are position in the experiment's axis system and the GPS coordinates, and the object's absolute velocity and compass heading.
      |
      | For more information, please click Help.
      settings: DeleteFcn=PreScanBlockDeleteFcn;
      mask Help: eval('openHelp(462)')
      mask Display:
      | port_label('output',1,'x [m]')
      | port_label('output',2,'y [m]')
      | port_label('output',3,'z [m]','texmode','on')
      | port_label('output',4,'Rotx [deg]','texmode','on')
      | port_label('output',5,'Roty [deg]','texmode','on')
      | port_label('output',6,'Rotz [deg]','texmode','on')
      | port_label('output',7,'GPS lat [deg]','texmode','on')
      | port_label('output',8,'GPS long [deg]','texmode','on')
      | port_label('output',9,'GPS alt [m]','texmode','on')
      | port_label('output',10,'Velocity [m/s]')
      | port_label('output',11,'Heading [deg]')
      | port_label('output',12,'Yaw rate [deg/s]')
      | port_label('output',13,'Timestamp [s]')
  STATE_Audi_A3_5_rc : RateTransition  Tag=mux_rc/StatePort  OutPortSampleTimeOpt=Inherit
  Terminator_{1..20} (20 alike) : Terminator
  STATE_Audi_A3_5_bus : Outport  Tag=outport/StatePort  OutDataTypeStr=Bus: PRESCAN_STATEACTUATORDATA  PortDimensions=1  SampleTime=1/20
  wires:
  STATE_Audi_A3_5_rc/1 -> STATE_Audi_A3_5_bus/1
  SELF_Audi_A3_5/1 -> SELF_Demux/1(SELF)
  AIR_9/1 -> AIR_9_Demux/1(AIR)
  Dynamics_Empty/1(State) -> STATE_Audi_A3_5_rc/1
  AIR_9_Demux/1(Range [m]) -> Terminator_1/1
  AIR_9_Demux/2(Azimuth [deg]) -> Terminator_2/1
  AIR_9_Demux/3(Elevation [deg]) -> Terminator_3/1
  AIR_9_Demux/4(ID [-]) -> Terminator_4/1
  AIR_9_Demux/5(Velocity [m/s]) -> Terminator_5/1
  AIR_9_Demux/6(Heading [deg]) -> Terminator_6/1
  AIR_9_Demux/7(Timestamp [s]) -> Terminator_7/1
  SELF_Demux/1(x [m]) -> Terminator_8/1
  SELF_Demux/2(y [m]) -> Terminator_9/1
  SELF_Demux/3(z [m]) -> Terminator_10/1
  SELF_Demux/4(rotx [deg]) -> Terminator_11/1
  SELF_Demux/5(roty [deg]) -> Terminator_12/1
  SELF_Demux/6(rotz [deg]) -> Terminator_13/1
  SELF_Demux/7(GPS lat [deg]) -> Terminator_14/1
  SELF_Demux/8(GPS long [deg]) -> Terminator_15/1
  SELF_Demux/9(GPS alt [m]) -> Terminator_16/1
  SELF_Demux/10(velocity [m/s]) -> Terminator_17/1
  SELF_Demux/11(heading [deg]) -> Terminator_18/1
  SELF_Demux/12(yaw rate [deg/s]) -> Terminator_19/1
  SELF_Demux/13(TimeStamp [s]) -> Terminator_20/1

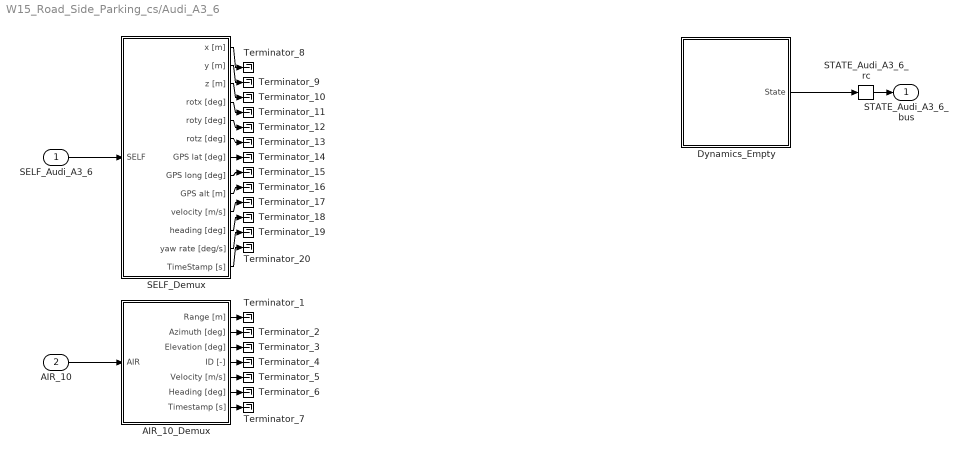
== system W15_Road_Side_Parking_cs/Audi_A3_6 ==
  SELF_Audi_A3_6 : Inport  Tag=inport/SelfPort  OutDataTypeStr=Bus: PRESCAN_SELFSENSORDATA  PortDimensions=1  SampleTime=1/20  BusOutputAsStruct=on
  AIR_10 : Inport  Tag=inport/AIR  Port=2  OutDataTypeStr=Bus: PRESCAN_AIRSENSORMESSAGE  PortDimensions=1  SampleTime=1/20  BusOutputAsStruct=on
  AIR_10_Demux : Subsystem  Tag=demux/AIR  mask(PreScan Demux Block: AIR){DetectionType=BBox, detectableObjects=1}
      mask prompts: DetectionType "Detection Type"; detectableObjects "Max. detectable objects"
      mask help:
      | The Actor Information Receiver sensor provides a fast, simple and generic detection solution which is not tied up to a specific technology and can be used for scenarios in which a simple sensor is needed.
      |
      | For more information, please click Help.
      mask init: same as W15_Road_Side_Parking_cs/Audi_A3_1/AIR_1_Demux
      settings: DeleteFcn=PreScanBlockDeleteFcn;
      mask Help: eval('openHelp(413)')
      mask TypeOptions DetectionType: Center | BBox | CoG
      mask Display:
      | disp(char('Det. type:         ',['{\it',DetectionTypeStr,'}']),'texmode','on')
      | port_label('output',1,'Range [m]')
      | port_label('output',2,'{\theta} [deg]','texmode','on')
      | port_label('output',3,'{\phi} [deg]','texmode','on')
      | port_label('output',4,'ID [-]','texmode','on')
      | port_label('output',5,'Velocity [m/s]','texmode','on')
      | port_label('output',6,'Heading [deg]','texmode','on')
      | port_label('output',7,'Timestamp [s]','texmode','on')
  Dynamics_Empty : Subsystem  Tag=Dynamics_Empty
      mask Help: eval('openHelp(202)')
      mask Display: port_label('output', 1, 'State');text(0,0,' Empty\n')
  SELF_Demux : Subsystem  Tag=demux/SelfPort  mask(PreScan Demux Block:){}
      mask help:
      | The SELF port shows (state) information of the actor itself. The outputs are position in the experiment's axis system and the GPS coordinates, and the object's absolute velocity and compass heading.
      |
      | For more information, please click Help.
      settings: DeleteFcn=PreScanBlockDeleteFcn;
      mask Help: eval('openHelp(462)')
      mask Display:
      | port_label('output',1,'x [m]')
      | port_label('output',2,'y [m]')
      | port_label('output',3,'z [m]','texmode','on')
      | port_label('output',4,'Rotx [deg]','texmode','on')
      | port_label('output',5,'Roty [deg]','texmode','on')
      | port_label('output',6,'Rotz [deg]','texmode','on')
      | port_label('output',7,'GPS lat [deg]','texmode','on')
      | port_label('output',8,'GPS long [deg]','texmode','on')
      | port_label('output',9,'GPS alt [m]','texmode','on')
      | port_label('output',10,'Velocity [m/s]')
      | port_label('output',11,'Heading [deg]')
      | port_label('output',12,'Yaw rate [deg/s]')
      | port_label('output',13,'Timestamp [s]')
  STATE_Audi_A3_6_rc : RateTransition  Tag=mux_rc/StatePort  OutPortSampleTimeOpt=Inherit
  Terminator_{1..20} (20 alike) : Terminator
  STATE_Audi_A3_6_bus : Outport  Tag=outport/StatePort  OutDataTypeStr=Bus: PRESCAN_STATEACTUATORDATA  PortDimensions=1  SampleTime=1/20
  wires:
  STATE_Audi_A3_6_rc/1 -> STATE_Audi_A3_6_bus/1
  SELF_Audi_A3_6/1 -> SELF_Demux/1(SELF)
  AIR_10/1 -> AIR_10_Demux/1(AIR)
  Dynamics_Empty/1(State) -> STATE_Audi_A3_6_rc/1
  AIR_10_Demux/1(Range [m]) -> Terminator_1/1
  AIR_10_Demux/2(Azimuth [deg]) -> Terminator_2/1
  AIR_10_Demux/3(Elevation [deg]) -> Terminator_3/1
  AIR_10_Demux/4(ID [-]) -> Terminator_4/1
  AIR_10_Demux/5(Velocity [m/s]) -> Terminator_5/1
  AIR_10_Demux/6(Heading [deg]) -> Terminator_6/1
  AIR_10_Demux/7(Timestamp [s]) -> Terminator_7/1
  SELF_Demux/1(x [m]) -> Terminator_8/1
  SELF_Demux/2(y [m]) -> Terminator_9/1
  SELF_Demux/3(z [m]) -> Terminator_10/1
  SELF_Demux/4(rotx [deg]) -> Terminator_11/1
  SELF_Demux/5(roty [deg]) -> Terminator_12/1
  SELF_Demux/6(rotz [deg]) -> Terminator_13/1
  SELF_Demux/7(GPS lat [deg]) -> Terminator_14/1
  SELF_Demux/8(GPS long [deg]) -> Terminator_15/1
  SELF_Demux/9(GPS alt [m]) -> Terminator_16/1
  SELF_Demux/10(velocity [m/s]) -> Terminator_17/1
  SELF_Demux/11(heading [deg]) -> Terminator_18/1
  SELF_Demux/12(yaw rate [deg/s]) -> Terminator_19/1
  SELF_Demux/13(TimeStamp [s]) -> Terminator_20/1

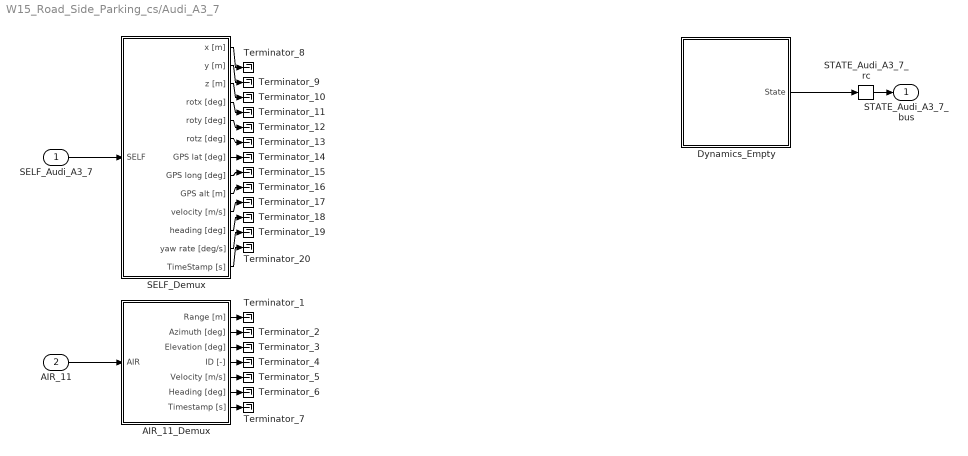
== system W15_Road_Side_Parking_cs/Audi_A3_7 ==
  SELF_Audi_A3_7 : Inport  Tag=inport/SelfPort  OutDataTypeStr=Bus: PRESCAN_SELFSENSORDATA  PortDimensions=1  SampleTime=1/20  BusOutputAsStruct=on
  AIR_11 : Inport  Tag=inport/AIR  Port=2  OutDataTypeStr=Bus: PRESCAN_AIRSENSORMESSAGE  PortDimensions=1  SampleTime=1/20  BusOutputAsStruct=on
  AIR_11_Demux : Subsystem  Tag=demux/AIR  mask(PreScan Demux Block: AIR){DetectionType=BBox, detectableObjects=1}
      mask prompts: DetectionType "Detection Type"; detectableObjects "Max. detectable objects"
      mask help:
      | The Actor Information Receiver sensor provides a fast, simple and generic detection solution which is not tied up to a specific technology and can be used for scenarios in which a simple sensor is needed.
      |
      | For more information, please click Help.
      mask init: same as W15_Road_Side_Parking_cs/Audi_A3_1/AIR_1_Demux
      settings: DeleteFcn=PreScanBlockDeleteFcn;
      mask Help: eval('openHelp(413)')
      mask TypeOptions DetectionType: Center | BBox | CoG
      mask Display:
      | disp(char('Det. type:         ',['{\it',DetectionTypeStr,'}']),'texmode','on')
      | port_label('output',1,'Range [m]')
      | port_label('output',2,'{\theta} [deg]','texmode','on')
      | port_label('output',3,'{\phi} [deg]','texmode','on')
      | port_label('output',4,'ID [-]','texmode','on')
      | port_label('output',5,'Velocity [m/s]','texmode','on')
      | port_label('output',6,'Heading [deg]','texmode','on')
      | port_label('output',7,'Timestamp [s]','texmode','on')
  Dynamics_Empty : Subsystem  Tag=Dynamics_Empty
      mask Help: eval('openHelp(202)')
      mask Display: port_label('output', 1, 'State');text(0,0,' Empty\n')
  SELF_Demux : Subsystem  Tag=demux/SelfPort  mask(PreScan Demux Block:){}
      mask help:
      | The SELF port shows (state) information of the actor itself. The outputs are position in the experiment's axis system and the GPS coordinates, and the object's absolute velocity and compass heading.
      |
      | For more information, please click Help.
      settings: DeleteFcn=PreScanBlockDeleteFcn;
      mask Help: eval('openHelp(462)')
      mask Display:
      | port_label('output',1,'x [m]')
      | port_label('output',2,'y [m]')
      | port_label('output',3,'z [m]','texmode','on')
      | port_label('output',4,'Rotx [deg]','texmode','on')
      | port_label('output',5,'Roty [deg]','texmode','on')
      | port_label('output',6,'Rotz [deg]','texmode','on')
      | port_label('output',7,'GPS lat [deg]','texmode','on')
      | port_label('output',8,'GPS long [deg]','texmode','on')
      | port_label('output',9,'GPS alt [m]','texmode','on')
      | port_label('output',10,'Velocity [m/s]')
      | port_label('output',11,'Heading [deg]')
      | port_label('output',12,'Yaw rate [deg/s]')
      | port_label('output',13,'Timestamp [s]')
  STATE_Audi_A3_7_rc : RateTransition  Tag=mux_rc/StatePort  OutPortSampleTimeOpt=Inherit
  Terminator_{1..20} (20 alike) : Terminator
  STATE_Audi_A3_7_bus : Outport  Tag=outport/StatePort  OutDataTypeStr=Bus: PRESCAN_STATEACTUATORDATA  PortDimensions=1  SampleTime=1/20
  wires:
  STATE_Audi_A3_7_rc/1 -> STATE_Audi_A3_7_bus/1
  SELF_Audi_A3_7/1 -> SELF_Demux/1(SELF)
  AIR_11/1 -> AIR_11_Demux/1(AIR)
  Dynamics_Empty/1(State) -> STATE_Audi_A3_7_rc/1
  AIR_11_Demux/1(Range [m]) -> Terminator_1/1
  AIR_11_Demux/2(Azimuth [deg]) -> Terminator_2/1
  AIR_11_Demux/3(Elevation [deg]) -> Terminator_3/1
  AIR_11_Demux/4(ID [-]) -> Terminator_4/1
  AIR_11_Demux/5(Velocity [m/s]) -> Terminator_5/1
  AIR_11_Demux/6(Heading [deg]) -> Terminator_6/1
  AIR_11_Demux/7(Timestamp [s]) -> Terminator_7/1
  SELF_Demux/1(x [m]) -> Terminator_8/1
  SELF_Demux/2(y [m]) -> Terminator_9/1
  SELF_Demux/3(z [m]) -> Terminator_10/1
  SELF_Demux/4(rotx [deg]) -> Terminator_11/1
  SELF_Demux/5(roty [deg]) -> Terminator_12/1
  SELF_Demux/6(rotz [deg]) -> Terminator_13/1
  SELF_Demux/7(GPS lat [deg]) -> Terminator_14/1
  SELF_Demux/8(GPS long [deg]) -> Terminator_15/1
  SELF_Demux/9(GPS alt [m]) -> Terminator_16/1
  SELF_Demux/10(velocity [m/s]) -> Terminator_17/1
  SELF_Demux/11(heading [deg]) -> Terminator_18/1
  SELF_Demux/12(yaw rate [deg/s]) -> Terminator_19/1
  SELF_Demux/13(TimeStamp [s]) -> Terminator_20/1

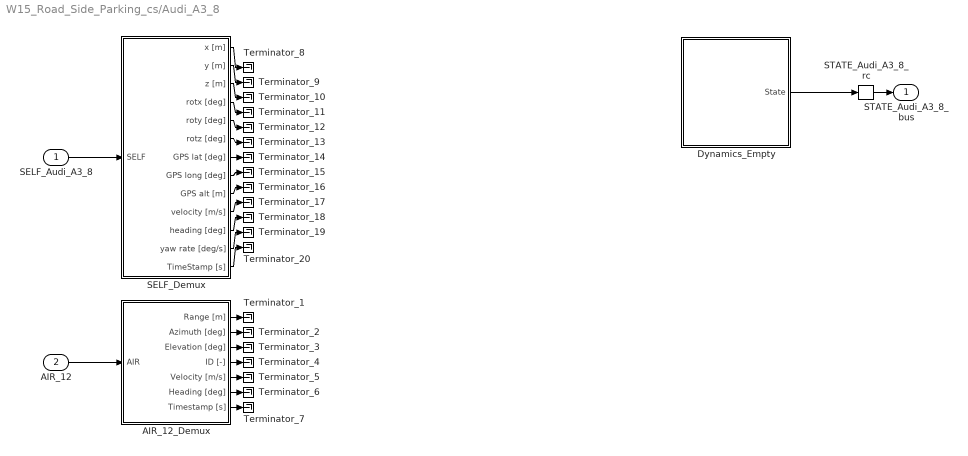
== system W15_Road_Side_Parking_cs/Audi_A3_8 ==
  SELF_Audi_A3_8 : Inport  Tag=inport/SelfPort  OutDataTypeStr=Bus: PRESCAN_SELFSENSORDATA  PortDimensions=1  SampleTime=1/20  BusOutputAsStruct=on
  AIR_12 : Inport  Tag=inport/AIR  Port=2  OutDataTypeStr=Bus: PRESCAN_AIRSENSORMESSAGE  PortDimensions=1  SampleTime=1/20  BusOutputAsStruct=on
  AIR_12_Demux : Subsystem  Tag=demux/AIR  mask(PreScan Demux Block: AIR){DetectionType=BBox, detectableObjects=1}
      mask prompts: DetectionType "Detection Type"; detectableObjects "Max. detectable objects"
      mask help:
      | The Actor Information Receiver sensor provides a fast, simple and generic detection solution which is not tied up to a specific technology and can be used for scenarios in which a simple sensor is needed.
      |
      | For more information, please click Help.
      mask init: same as W15_Road_Side_Parking_cs/Audi_A3_1/AIR_1_Demux
      settings: DeleteFcn=PreScanBlockDeleteFcn;
      mask Help: eval('openHelp(413)')
      mask TypeOptions DetectionType: Center | BBox | CoG
      mask Display:
      | disp(char('Det. type:         ',['{\it',DetectionTypeStr,'}']),'texmode','on')
      | port_label('output',1,'Range [m]')
      | port_label('output',2,'{\theta} [deg]','texmode','on')
      | port_label('output',3,'{\phi} [deg]','texmode','on')
      | port_label('output',4,'ID [-]','texmode','on')
      | port_label('output',5,'Velocity [m/s]','texmode','on')
      | port_label('output',6,'Heading [deg]','texmode','on')
      | port_label('output',7,'Timestamp [s]','texmode','on')
  Dynamics_Empty : Subsystem  Tag=Dynamics_Empty
      mask Help: eval('openHelp(202)')
      mask Display: port_label('output', 1, 'State');text(0,0,' Empty\n')
  SELF_Demux : Subsystem  Tag=demux/SelfPort  mask(PreScan Demux Block:){}
      mask help:
      | The SELF port shows (state) information of the actor itself. The outputs are position in the experiment's axis system and the GPS coordinates, and the object's absolute velocity and compass heading.
      |
      | For more information, please click Help.
      settings: DeleteFcn=PreScanBlockDeleteFcn;
      mask Help: eval('openHelp(462)')
      mask Display:
      | port_label('output',1,'x [m]')
      | port_label('output',2,'y [m]')
      | port_label('output',3,'z [m]','texmode','on')
      | port_label('output',4,'Rotx [deg]','texmode','on')
      | port_label('output',5,'Roty [deg]','texmode','on')
      | port_label('output',6,'Rotz [deg]','texmode','on')
      | port_label('output',7,'GPS lat [deg]','texmode','on')
      | port_label('output',8,'GPS long [deg]','texmode','on')
      | port_label('output',9,'GPS alt [m]','texmode','on')
      | port_label('output',10,'Velocity [m/s]')
      | port_label('output',11,'Heading [deg]')
      | port_label('output',12,'Yaw rate [deg/s]')
      | port_label('output',13,'Timestamp [s]')
  STATE_Audi_A3_8_rc : RateTransition  Tag=mux_rc/StatePort  OutPortSampleTimeOpt=Inherit
  Terminator_{1..20} (20 alike) : Terminator
  STATE_Audi_A3_8_bus : Outport  Tag=outport/StatePort  OutDataTypeStr=Bus: PRESCAN_STATEACTUATORDATA  PortDimensions=1  SampleTime=1/20
  wires:
  STATE_Audi_A3_8_rc/1 -> STATE_Audi_A3_8_bus/1
  SELF_Audi_A3_8/1 -> SELF_Demux/1(SELF)
  AIR_12/1 -> AIR_12_Demux/1(AIR)
  Dynamics_Empty/1(State) -> STATE_Audi_A3_8_rc/1
  AIR_12_Demux/1(Range [m]) -> Terminator_1/1
  AIR_12_Demux/2(Azimuth [deg]) -> Terminator_2/1
  AIR_12_Demux/3(Elevation [deg]) -> Terminator_3/1
  AIR_12_Demux/4(ID [-]) -> Terminator_4/1
  AIR_12_Demux/5(Velocity [m/s]) -> Terminator_5/1
  AIR_12_Demux/6(Heading [deg]) -> Terminator_6/1
  AIR_12_Demux/7(Timestamp [s]) -> Terminator_7/1
  SELF_Demux/1(x [m]) -> Terminator_8/1
  SELF_Demux/2(y [m]) -> Terminator_9/1
  SELF_Demux/3(z [m]) -> Terminator_10/1
  SELF_Demux/4(rotx [deg]) -> Terminator_11/1
  SELF_Demux/5(roty [deg]) -> Terminator_12/1
  SELF_Demux/6(rotz [deg]) -> Terminator_13/1
  SELF_Demux/7(GPS lat [deg]) -> Terminator_14/1
  SELF_Demux/8(GPS long [deg]) -> Terminator_15/1
  SELF_Demux/9(GPS alt [m]) -> Terminator_16/1
  SELF_Demux/10(velocity [m/s]) -> Terminator_17/1
  SELF_Demux/11(heading [deg]) -> Terminator_18/1
  SELF_Demux/12(yaw rate [deg/s]) -> Terminator_19/1
  SELF_Demux/13(TimeStamp [s]) -> Terminator_20/1

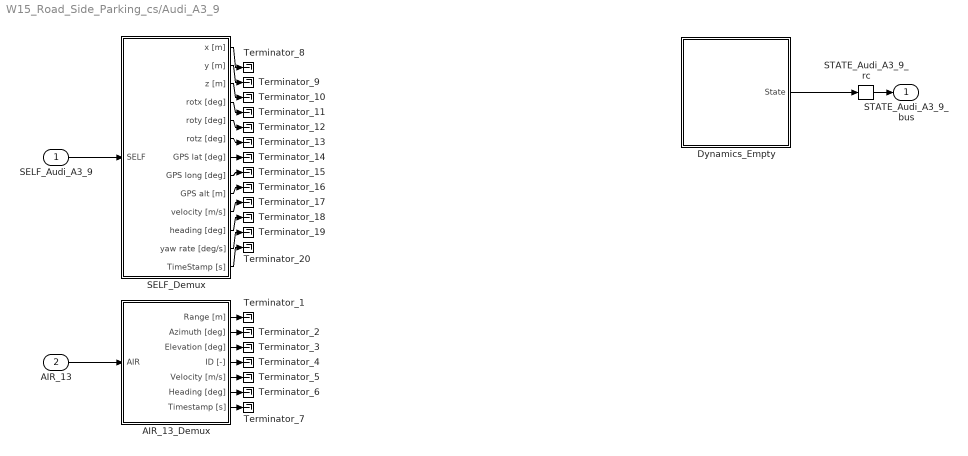
== system W15_Road_Side_Parking_cs/Audi_A3_9 ==
  SELF_Audi_A3_9 : Inport  Tag=inport/SelfPort  OutDataTypeStr=Bus: PRESCAN_SELFSENSORDATA  PortDimensions=1  SampleTime=1/20  BusOutputAsStruct=on
  AIR_13 : Inport  Tag=inport/AIR  Port=2  OutDataTypeStr=Bus: PRESCAN_AIRSENSORMESSAGE  PortDimensions=1  SampleTime=1/20  BusOutputAsStruct=on
  AIR_13_Demux : Subsystem  Tag=demux/AIR  mask(PreScan Demux Block: AIR){DetectionType=BBox, detectableObjects=1}
      mask prompts: DetectionType "Detection Type"; detectableObjects "Max. detectable objects"
      mask help:
      | The Actor Information Receiver sensor provides a fast, simple and generic detection solution which is not tied up to a specific technology and can be used for scenarios in which a simple sensor is needed.
      |
      | For more information, please click Help.
      mask init: same as W15_Road_Side_Parking_cs/Audi_A3_1/AIR_1_Demux
      settings: DeleteFcn=PreScanBlockDeleteFcn;
      mask Help: eval('openHelp(413)')
      mask TypeOptions DetectionType: Center | BBox | CoG
      mask Display:
      | disp(char('Det. type:         ',['{\it',DetectionTypeStr,'}']),'texmode','on')
      | port_label('output',1,'Range [m]')
      | port_label('output',2,'{\theta} [deg]','texmode','on')
      | port_label('output',3,'{\phi} [deg]','texmode','on')
      | port_label('output',4,'ID [-]','texmode','on')
      | port_label('output',5,'Velocity [m/s]','texmode','on')
      | port_label('output',6,'Heading [deg]','texmode','on')
      | port_label('output',7,'Timestamp [s]','texmode','on')
  Dynamics_Empty : Subsystem  Tag=Dynamics_Empty
      mask Help: eval('openHelp(202)')
      mask Display: port_label('output', 1, 'State');text(0,0,' Empty\n')
  SELF_Demux : Subsystem  Tag=demux/SelfPort  mask(PreScan Demux Block:){}
      mask help:
      | The SELF port shows (state) information of the actor itself. The outputs are position in the experiment's axis system and the GPS coordinates, and the object's absolute velocity and compass heading.
      |
      | For more information, please click Help.
      settings: DeleteFcn=PreScanBlockDeleteFcn;
      mask Help: eval('openHelp(462)')
      mask Display:
      | port_label('output',1,'x [m]')
      | port_label('output',2,'y [m]')
      | port_label('output',3,'z [m]','texmode','on')
      | port_label('output',4,'Rotx [deg]','texmode','on')
      | port_label('output',5,'Roty [deg]','texmode','on')
      | port_label('output',6,'Rotz [deg]','texmode','on')
      | port_label('output',7,'GPS lat [deg]','texmode','on')
      | port_label('output',8,'GPS long [deg]','texmode','on')
      | port_label('output',9,'GPS alt [m]','texmode','on')
      | port_label('output',10,'Velocity [m/s]')
      | port_label('output',11,'Heading [deg]')
      | port_label('output',12,'Yaw rate [deg/s]')
      | port_label('output',13,'Timestamp [s]')
  STATE_Audi_A3_9_rc : RateTransition  Tag=mux_rc/StatePort  OutPortSampleTimeOpt=Inherit
  Terminator_{1..20} (20 alike) : Terminator
  STATE_Audi_A3_9_bus : Outport  Tag=outport/StatePort  OutDataTypeStr=Bus: PRESCAN_STATEACTUATORDATA  PortDimensions=1  SampleTime=1/20
  wires:
  STATE_Audi_A3_9_rc/1 -> STATE_Audi_A3_9_bus/1
  SELF_Audi_A3_9/1 -> SELF_Demux/1(SELF)
  AIR_13/1 -> AIR_13_Demux/1(AIR)
  Dynamics_Empty/1(State) -> STATE_Audi_A3_9_rc/1
  AIR_13_Demux/1(Range [m]) -> Terminator_1/1
  AIR_13_Demux/2(Azimuth [deg]) -> Terminator_2/1
  AIR_13_Demux/3(Elevation [deg]) -> Terminator_3/1
  AIR_13_Demux/4(ID [-]) -> Terminator_4/1
  AIR_13_Demux/5(Velocity [m/s]) -> Terminator_5/1
  AIR_13_Demux/6(Heading [deg]) -> Terminator_6/1
  AIR_13_Demux/7(Timestamp [s]) -> Terminator_7/1
  SELF_Demux/1(x [m]) -> Terminator_8/1
  SELF_Demux/2(y [m]) -> Terminator_9/1
  SELF_Demux/3(z [m]) -> Terminator_10/1
  SELF_Demux/4(rotx [deg]) -> Terminator_11/1
  SELF_Demux/5(roty [deg]) -> Terminator_12/1
  SELF_Demux/6(rotz [deg]) -> Terminator_13/1
  SELF_Demux/7(GPS lat [deg]) -> Terminator_14/1
  SELF_Demux/8(GPS long [deg]) -> Terminator_15/1
  SELF_Demux/9(GPS alt [m]) -> Terminator_16/1
  SELF_Demux/10(velocity [m/s]) -> Terminator_17/1
  SELF_Demux/11(heading [deg]) -> Terminator_18/1
  SELF_Demux/12(yaw rate [deg/s]) -> Terminator_19/1
  SELF_Demux/13(TimeStamp [s]) -> Terminator_20/1
